simulink model "mpc_controller"  (R2019b)
settings: Solver=VariableStepAuto  StartTime=0.0  StopTime=10.0  RelTol=1e-3
libraries: mpcadaslib x1
settings Model: Creator=senoa95  LastModifiedBy=senoa95

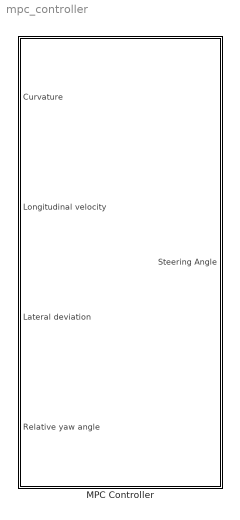
== system mpc_controller ==
  "MPC Controller " : Subsystem

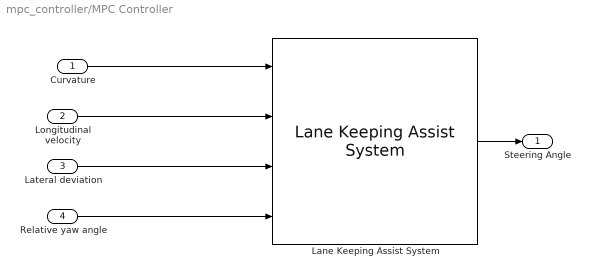
== system mpc_controller/MPC Controller  ==
  Curvature : Inport
  Longitudinal velocity : Inport  Port=2
  Lateral deviation : Inport  Port=3
  Relative yaw angle : Inport  Port=4
  Lane Keeping Assist System : mpcadaslib/Lane Keeping Assist System  ModelType=Use vehicle parameters  VehicleMass=1575  VehicleYawInertia=2875  LengthToFront=1.2  LengthToRear=1.6  FrontTireStiffness=19000  RearTireStiffness=33000  EgoModelMatrixA=[-4.4021 ,-12.4603;1.3913,-5.1868]  EgoModelMatrixB=[24.1270;15.8609]  EgoModelMatrixC=[1,0;0,1]  InitialLongVel=15  TransportLag=0  MinSteering=-0.26  umin_ext=off  MaxSteering=0.26  umax_ext=off  Ts=0.1  PredictionHorizon=10  ControllerBehavior=0.5  suboptimal=off  maxiter=10  datatypeopt=double  optmode=off  trackmode=off
      settings: SourceProductName=Model Predictive Control Toolbox  SourceProductBaseCode=MP
  Steering Angle : Outport  VectorParamsAs1DForOutWhenUnconnected=off
  wires:
  Lane Keeping Assist System/1 -> Steering Angle/1
  Curvature/1 -> Lane Keeping Assist System/1
  Longitudinal velocity/1 -> Lane Keeping Assist System/2
  Lateral deviation/1 -> Lane Keeping Assist System/3
  Relative yaw angle/1 -> Lane Keeping Assist System/4
